simulink model "InportShadow"  (R2017b)
settings: Solver=FixedStepDiscrete  StartTime=0.0  StopTime=10.0  FixedStep=0.200000  RelTol=1e-3
settings Model: Creator=hbourbou  LastModifiedBy=hbourbou
settings DataIOCC: SaveFormat=StructureWithTime
settings OptimizationCC: LifeSpan=inf
settings DebuggingCC: SFExecutionAtInitializationDiag=none
settings HardwareCC: ProdBitPerSizeT=32  ProdBitPerPtrDiffT=32  ProdWordSize=32  ProdHWDeviceType=Specified
settings CodeAppCC: StateflowObjectComments=on

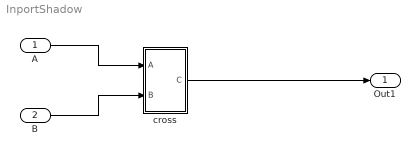
== system InportShadow ==
  A : Inport
  B : Inport  Port=2
  cross : Subsystem
  Out1 : Outport  OutMin=1  OutMax=5
  wires:
  cross/1(C) -> Out1/1
  A/1 -> cross/1(A)
  B/1 -> cross/2(B)

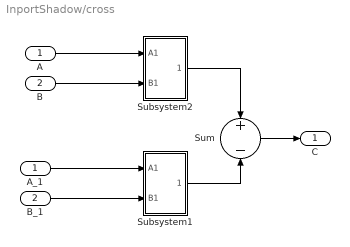
== system InportShadow/cross ==
  A : Inport
  B : Inport  Port=2
  A_1 : InportShadow
  B_1 : InportShadow  Port=2
  Subsystem1 : Subsystem
  Subsystem2 : Subsystem
  Sum : Sum  Inputs=+|-  SaturateOnIntegerOverflow=on  InputSameDT=on  OutDataTypeStr=Inherit: Same as first input
  C : Outport
  wires:
  B/1 -> Subsystem2/2(B1)
  A/1 -> Subsystem2/1(A1)
  Subsystem2/1(Out1) -> Sum/1
  Sum/1 -> C/1
  Subsystem1/1(Out1) -> Sum/2
  A_1/1 -> Subsystem1/1(A1)
  B_1/1 -> Subsystem1/2(B1)

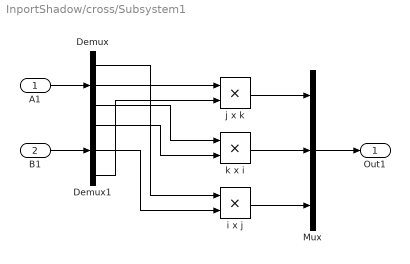
== system InportShadow/cross/Subsystem1 ==
  A1 : Inport
  B1 : Inport  Port=2
  Demux : Demux  Outputs=3
  Demux1 : Demux  Outputs=3
  Mux : Mux  Inputs=3
  i x j : Product  SaturateOnIntegerOverflow=on  InputSameDT=on  OutDataTypeStr=Inherit: Same as first input
  j x k : Product  SaturateOnIntegerOverflow=on  InputSameDT=on  OutDataTypeStr=Inherit: Same as first input
  k x i : Product  SaturateOnIntegerOverflow=on  InputSameDT=on  OutDataTypeStr=Inherit: Same as first input
  Out1 : Outport
  wires:
  Demux/2 -> j x k/1
  Demux1/3 -> j x k/2
  A1/1 -> Demux/1
  Demux/3 -> k x i/1
  Mux/1 -> Out1/1
  j x k/1 -> Mux/1
  B1/1 -> Demux1/1
  k x i/1 -> Mux/2
  Demux1/2 -> i x j/2
  i x j/1 -> Mux/3
  Demux/1 -> i x j/1
  Demux1/1 -> k x i/2

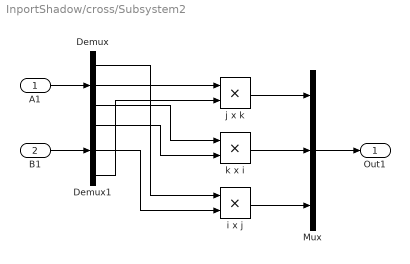
== system InportShadow/cross/Subsystem2 ==
  A1 : Inport
  B1 : Inport  Port=2
  Demux : Demux  Outputs=3
  Demux1 : Demux  Outputs=3
  Mux : Mux  Inputs=3
  i x j : Product  SaturateOnIntegerOverflow=on  InputSameDT=on  OutDataTypeStr=Inherit: Same as first input
  j x k : Product  SaturateOnIntegerOverflow=on  InputSameDT=on  OutDataTypeStr=Inherit: Same as first input
  k x i : Product  SaturateOnIntegerOverflow=on  InputSameDT=on  OutDataTypeStr=Inherit: Same as first input
  Out1 : Outport
  wires:
  Demux1/1 -> k x i/2
  Demux/1 -> i x j/1
  i x j/1 -> Mux/3
  Demux1/2 -> i x j/2
  k x i/1 -> Mux/2
  B1/1 -> Demux1/1
  j x k/1 -> Mux/1
  Mux/1 -> Out1/1
  Demux/3 -> k x i/1
  A1/1 -> Demux/1
  Demux1/3 -> j x k/2
  Demux/2 -> j x k/1
